simulink model "P702_NI_SoftECU"  (R2019a)
settings: Solver=ode1  StartTime=0.0  StopTime=Inf  FixedStep=0.001  RelTol=1e-3  EnableMultiTasking=on
PreLoadFcn:
  | run '.\VeriStand_BlockSet\NIVeriStandAddPaths.m'
undefined symbols (not defined in the file or in its folder): magnitude
libraries: simulink x83, simulink_extras x1
(part 70 of 76)

== system P702_NI_SoftECU/SoftECU/SRR_L/FrontLeft_SOD/SRR_FL_002/Subsystem ==
  target_pos : Inport
  sensor_pos : Inport  Port=2
  CSP : Inport  Port=3
  Abs : Abs
  Add : Sum  Inputs=++-+
  Add1 : Sum  Inputs=++-+
  Add2 : Sum  Inputs=+-
  Add3 : Sum
  Bus Selector : BusSelector  OutputSignals=SRR_L_DET_RANGE_02[m],SRR_L_DET_AZIMUTH_02[rad],SRR_L_DET_RANGE_RATE_02[m/s],SRR_L_DET_ELEVATION_02[rad]
  Bus Selector1 : BusSelector  OutputSignals=sensor_x,sensor_y,sensor_yaw
  Bus Selector2 : BusSelector  OutputSignals=c_sensor_x,c_sensor_y,c_sensor_yaw
  Constant : Constant
  Index Vector : MultiPortSwitch  DataPortOrder=Zero-based contiguous  Inputs=2  zeroidx=on
  Index Vector1 : MultiPortSwitch  DataPortOrder=Zero-based contiguous  Inputs=2  zeroidx=on
  Logical Operator : Logic  AllPortsSameDT=off  OutDataTypeStr=boolean
  Math Function : Math  Operator=magnitude^2  SaturateOnIntegerOverflow=on
  Math Function1 : Math  Operator=magnitude^2  SaturateOnIntegerOverflow=on
  Product : Product
  Product1 : Product
  Product2 : Product
  Relational Operator : RelationalOperator  Operator=<=  OutDataTypeStr=boolean  RndMeth=Simplest
  Relational Operator1 : RelationalOperator  Operator=<=  OutDataTypeStr=boolean  RndMeth=Simplest
  Sqrt : Sqrt  SaturateOnIntegerOverflow=on
  Terminator : Terminator
  atan_cal : Trigonometry  Operator=atan2
  atan_cal1 : Trigonometry  Operator=atan2
  not_valid_azimuth : Constant  Value=0
  not_valid_range : Constant  Value=-1
  random_factor : Subsystem
  random_factor1 : Subsystem
  sincal : Trigonometry
  sincal1 : Trigonometry  Operator=cos
  sincal2 : Trigonometry
  sincal3 : Trigonometry  Operator=cos
  range : Outport
  range_rate : Outport  Port=2
  azimuth : Outport  Port=3
  elevation : Outport  Port=4
  wires:
  target_pos/1 -> Bus Selector/1
  Bus Selector/1 -> random_factor/1(Range), random_factor1/1(Range), Product1/1, Product/1  "<SRR_L_DET_RANGE_02[m]>"
  Bus Selector/2 -> sincal1/1, sincal/1  "<SRR_L_DET_AZIMUTH_02[rad]>"
  sincal/1 -> Product/2
  sincal1/1 -> Product1/2
  Product/1 -> Add/1
  sensor_pos/1 -> Bus Selector1/1
  CSP/1 -> Bus Selector2/1
  Bus Selector2/1 -> Add1/2  "<c_sensor_x>"
  Bus Selector2/2 -> Add/2  "<c_sensor_y>"
  Bus Selector2/3 -> Terminator/1  "<c_sensor_yaw>"
  Bus Selector1/1 -> Add1/3  "<sensor_x>"
  Bus Selector1/2 -> Add/3  "<sensor_y>"
  Bus Selector1/3 -> Add2/2  "<sensor_yaw>"
  Product1/1 -> Add1/1
  Add/1 -> Math Function/1, atan_cal/1
  Add1/1 -> Math Function1/1, atan_cal/2
  atan_cal/1 -> Add2/1
  Math Function/1 -> Add3/1
  Math Function1/1 -> Add3/2
  Add3/1 -> Sqrt/1
  Constant/1 -> Product2/2
  Bus Selector/3 -> range_rate/1  "<SRR_L_DET_RANGE_RATE_02[m/s]>"
  Bus Selector/4 -> elevation/1  "<SRR_L_DET_ELEVATION_02[rad]>"
  Sqrt/1 -> Index Vector/3, Relational Operator/1
  Product2/1 -> Abs/1, Index Vector1/3
  Relational Operator/1 -> Logical Operator/1
  Relational Operator1/1 -> Logical Operator/2
  Index Vector/1 -> range/1
  not_valid_range/1 -> Index Vector/2
  Index Vector1/1 -> azimuth/1
  Logical Operator/1 -> Index Vector1/1, Index Vector/1
  not_valid_azimuth/1 -> Index Vector1/2
  atan_cal1/1 -> Product2/1
  sincal2/1 -> atan_cal1/1
  sincal3/1 -> atan_cal1/2
  Add2/1 -> sincal3/1, sincal2/1
  Abs/1 -> Relational Operator1/1
  [DistanceScanRange] -> Relational Operator/2
  [AngleScanRange] -> Relational Operator1/2
  random_factor/1(Rand_Error) -> Add/4
  random_factor1/1(Rand_Error) -> Add1/4

== system P702_NI_SoftECU/SoftECU/SRR_L/FrontLeft_SOD/SRR_FL_003/Subsystem ==
  target_pos : Inport
  sensor_pos : Inport  Port=2
  CSP : Inport  Port=3
  Abs : Abs
  Add : Sum  Inputs=++-+
  Add1 : Sum  Inputs=++-+
  Add2 : Sum  Inputs=+-
  Add3 : Sum
  Bus Selector : BusSelector  OutputSignals=SRR_L_DET_RANGE_03[m],SRR_L_DET_AZIMUTH_03[rad],SRR_L_DET_RANGE_RATE_03[m/s],SRR_L_DET_ELEVATION_03[rad]
  Bus Selector1 : BusSelector  OutputSignals=sensor_x,sensor_y,sensor_yaw
  Bus Selector2 : BusSelector  OutputSignals=c_sensor_x,c_sensor_y,c_sensor_yaw
  Constant : Constant
  Index Vector : MultiPortSwitch  DataPortOrder=Zero-based contiguous  Inputs=2  zeroidx=on
  Index Vector1 : MultiPortSwitch  DataPortOrder=Zero-based contiguous  Inputs=2  zeroidx=on
  Logical Operator : Logic  AllPortsSameDT=off  OutDataTypeStr=boolean
  Math Function : Math  Operator=magnitude^2  SaturateOnIntegerOverflow=on
  Math Function1 : Math  Operator=magnitude^2  SaturateOnIntegerOverflow=on
  Product : Product
  Product1 : Product
  Product2 : Product
  Relational Operator : RelationalOperator  Operator=<=  OutDataTypeStr=boolean  RndMeth=Simplest
  Relational Operator1 : RelationalOperator  Operator=<=  OutDataTypeStr=boolean  RndMeth=Simplest
  Sqrt : Sqrt  SaturateOnIntegerOverflow=on
  Terminator : Terminator
  atan_cal : Trigonometry  Operator=atan2
  atan_cal1 : Trigonometry  Operator=atan2
  not_valid_azimuth : Constant  Value=0
  not_valid_range : Constant  Value=-1
  random_factor : Subsystem
  random_factor1 : Subsystem
  sincal : Trigonometry
  sincal1 : Trigonometry  Operator=cos
  sincal2 : Trigonometry
  sincal3 : Trigonometry  Operator=cos
  range : Outport
  range_rate : Outport  Port=2
  azimuth : Outport  Port=3
  elevation : Outport  Port=4
  wires:
  random_factor1/1(Rand_Error) -> Add1/4
  random_factor/1(Rand_Error) -> Add/4
  [AngleScanRange] -> Relational Operator1/2
  [DistanceScanRange] -> Relational Operator/2
  Abs/1 -> Relational Operator1/1
  Add2/1 -> sincal2/1, sincal3/1
  sincal3/1 -> atan_cal1/2
  sincal2/1 -> atan_cal1/1
  atan_cal1/1 -> Product2/1
  not_valid_azimuth/1 -> Index Vector1/2
  Logical Operator/1 -> Index Vector/1, Index Vector1/1
  Index Vector1/1 -> azimuth/1
  not_valid_range/1 -> Index Vector/2
  Index Vector/1 -> range/1
  Relational Operator1/1 -> Logical Operator/2
  Relational Operator/1 -> Logical Operator/1
  Product2/1 -> Index Vector1/3, Abs/1
  Sqrt/1 -> Relational Operator/1, Index Vector/3
  Bus Selector/4 -> elevation/1  "<SRR_L_DET_ELEVATION_03[rad]>"
  Bus Selector/3 -> range_rate/1  "<SRR_L_DET_RANGE_RATE_03[m/s]>"
  Constant/1 -> Product2/2
  Add3/1 -> Sqrt/1
  Math Function1/1 -> Add3/2
  Math Function/1 -> Add3/1
  atan_cal/1 -> Add2/1
  Add1/1 -> atan_cal/2, Math Function1/1
  Add/1 -> atan_cal/1, Math Function/1
  Product1/1 -> Add1/1
  Bus Selector1/3 -> Add2/2  "<sensor_yaw>"
  Bus Selector1/2 -> Add/3  "<sensor_y>"
  Bus Selector1/1 -> Add1/3  "<sensor_x>"
  Bus Selector2/3 -> Terminator/1  "<c_sensor_yaw>"
  Bus Selector2/2 -> Add/2  "<c_sensor_y>"
  Bus Selector2/1 -> Add1/2  "<c_sensor_x>"
  CSP/1 -> Bus Selector2/1
  sensor_pos/1 -> Bus Selector1/1
  Product/1 -> Add/1
  sincal1/1 -> Product1/2
  sincal/1 -> Product/2
  Bus Selector/2 -> sincal/1, sincal1/1  "<SRR_L_DET_AZIMUTH_03[rad]>"
  Bus Selector/1 -> Product/1, Product1/1, random_factor1/1(Range), random_factor/1(Range)  "<SRR_L_DET_RANGE_03[m]>"
  target_pos/1 -> Bus Selector/1

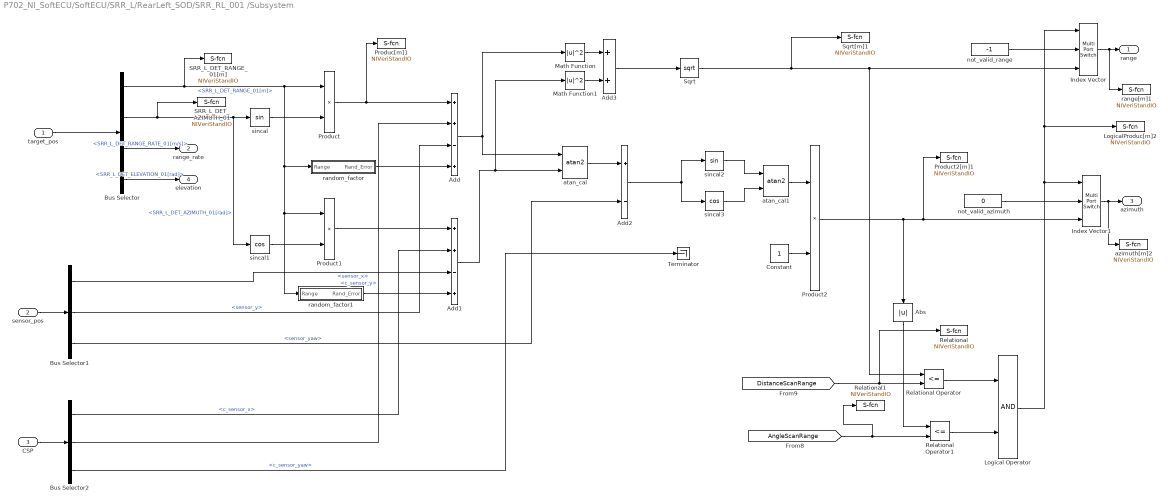
== system P702_NI_SoftECU/SoftECU/SRR_L/RearLeft_SOD/SRR_RL_001 /Subsystem ==
  target_pos : Inport
  sensor_pos : Inport  Port=2
  CSP : Inport  Port=3
  Abs : Abs
  Add : Sum  Inputs=++-+
  Add1 : Sum  Inputs=++-+
  Add2 : Sum  Inputs=+-
  Add3 : Sum
  Bus Selector : BusSelector  OutputSignals=SRR_L_DET_RANGE_01[m],SRR_L_DET_AZIMUTH_01[rad],SRR_L_DET_RANGE_RATE_01[m/s],SRR_L_DET_ELEVATION_01[rad]
  Bus Selector1 : BusSelector  OutputSignals=sensor_x,sensor_y,sensor_yaw
  Bus Selector2 : BusSelector  OutputSignals=c_sensor_x,c_sensor_y,c_sensor_yaw
  Constant : Constant
  Index Vector : MultiPortSwitch  DataPortOrder=Zero-based contiguous  Inputs=2  zeroidx=on
  Index Vector1 : MultiPortSwitch  DataPortOrder=Zero-based contiguous  Inputs=2  zeroidx=on
  Logical Operator : Logic  AllPortsSameDT=off  OutDataTypeStr=boolean
  LogicalProduc[m]2 : S-Function  Priority=4  FunctionName=NIVeriStandIO  Parameters=width dtype portnum stime stype btype  SFunctionDeploymentMode=off  EnableBusSupport=off  mask(NI VeriStand Outport){portnum=4, width=-1, stime=-1, dtype=auto, stype=auto, btype=0}
      mask prompts: portnum "Port number:"; width "Port dimensions (-1 for dynamically sized):"; stime "Sample time (-1 for inherited):"; dtype "Data type:"; stype "Signal type:"; btype "Block type:"
      mask help: Use this outport on any level of nested subsystems to allow NI VeriStand software to map signals to it.
      mask init:
      | NIVeriStandIO_init;
      settings: CopyFcn=NIVeriStand_MDL_functions('', 'IO_copy');  DeleteFcn=NIVeriStand_MDL_functions('', 'IO_delete');  MoveFcn=set_param(gcb, 'Mask', 'on');
      mask Callback portnum: NIVeriStand_MDL_functions('', 'IO_setportnum');
      mask TypeOptions dtype: auto | double | single | int8 | uint8 | int16 | uint16 | int32 | uint32 | boolean
      mask Callback dtype: NIVeriStand_MDL_functions('', 'IO_booleansignal');
      mask TypeOptions stype: auto | real | complex
      mask Display:
      | patch([-x x], [-y y], [.90980 .81960 .32156]);
      | plot([xrad -x x xrad], [yrad -y y yrad]);
      | fprintf('NI Out%d', portnum);
  Math Function : Math  Operator=magnitude^2  SaturateOnIntegerOverflow=on
  Math Function1 : Math  Operator=magnitude^2  SaturateOnIntegerOverflow=on
  Produc[m]1 : S-Function  Priority=3  FunctionName=NIVeriStandIO  Parameters=width dtype portnum stime stype btype  SFunctionDeploymentMode=off  EnableBusSupport=off  mask(NI VeriStand Outport){portnum=3, width=-1, stime=-1, dtype=auto, stype=auto, btype=0}
      mask prompts: portnum "Port number:"; width "Port dimensions (-1 for dynamically sized):"; stime "Sample time (-1 for inherited):"; dtype "Data type:"; stype "Signal type:"; btype "Block type:"
      mask help: Use this outport on any level of nested subsystems to allow NI VeriStand software to map signals to it.
      mask init:
      | NIVeriStandIO_init;
      settings: CopyFcn=NIVeriStand_MDL_functions('', 'IO_copy');  DeleteFcn=NIVeriStand_MDL_functions('', 'IO_delete');  MoveFcn=set_param(gcb, 'Mask', 'on');
      mask Callback portnum: NIVeriStand_MDL_functions('', 'IO_setportnum');
      mask TypeOptions dtype: auto | double | single | int8 | uint8 | int16 | uint16 | int32 | uint32 | boolean
      mask Callback dtype: NIVeriStand_MDL_functions('', 'IO_booleansignal');
      mask TypeOptions stype: auto | real | complex
      mask Display:
      | patch([-x x], [-y y], [.90980 .81960 .32156]);
      | plot([xrad -x x xrad], [yrad -y y yrad]);
      | fprintf('NI Out%d', portnum);
  Product : Product
  Product1 : Product
  Product2 : Product
  Product2[m]1 : S-Function  Priority=6  FunctionName=NIVeriStandIO  Parameters=width dtype portnum stime stype btype  SFunctionDeploymentMode=off  EnableBusSupport=off  mask(NI VeriStand Outport){portnum=6, width=-1, stime=-1, dtype=auto, stype=auto, btype=0}
      mask prompts: portnum "Port number:"; width "Port dimensions (-1 for dynamically sized):"; stime "Sample time (-1 for inherited):"; dtype "Data type:"; stype "Signal type:"; btype "Block type:"
      mask help: Use this outport on any level of nested subsystems to allow NI VeriStand software to map signals to it.
      mask init:
      | NIVeriStandIO_init;
      settings: CopyFcn=NIVeriStand_MDL_functions('', 'IO_copy');  DeleteFcn=NIVeriStand_MDL_functions('', 'IO_delete');  MoveFcn=set_param(gcb, 'Mask', 'on');
      mask Callback portnum: NIVeriStand_MDL_functions('', 'IO_setportnum');
      mask TypeOptions dtype: auto | double | single | int8 | uint8 | int16 | uint16 | int32 | uint32 | boolean
      mask Callback dtype: NIVeriStand_MDL_functions('', 'IO_booleansignal');
      mask TypeOptions stype: auto | real | complex
      mask Display:
      | patch([-x x], [-y y], [.90980 .81960 .32156]);
      | plot([xrad -x x xrad], [yrad -y y yrad]);
      | fprintf('NI Out%d', portnum);
  Relational : S-Function  Priority=7  FunctionName=NIVeriStandIO  Parameters=width dtype portnum stime stype btype  SFunctionDeploymentMode=off  EnableBusSupport=off  mask(NI VeriStand Outport){portnum=7, width=-1, stime=-1, dtype=auto, stype=auto, btype=0}
      mask prompts: portnum "Port number:"; width "Port dimensions (-1 for dynamically sized):"; stime "Sample time (-1 for inherited):"; dtype "Data type:"; stype "Signal type:"; btype "Block type:"
      mask help: Use this outport on any level of nested subsystems to allow NI VeriStand software to map signals to it.
      mask init:
      | NIVeriStandIO_init;
      settings: CopyFcn=NIVeriStand_MDL_functions('', 'IO_copy');  DeleteFcn=NIVeriStand_MDL_functions('', 'IO_delete');  MoveFcn=set_param(gcb, 'Mask', 'on');
      mask Callback portnum: NIVeriStand_MDL_functions('', 'IO_setportnum');
      mask TypeOptions dtype: auto | double | single | int8 | uint8 | int16 | uint16 | int32 | uint32 | boolean
      mask Callback dtype: NIVeriStand_MDL_functions('', 'IO_booleansignal');
      mask TypeOptions stype: auto | real | complex
      mask Display:
      | patch([-x x], [-y y], [.90980 .81960 .32156]);
      | plot([xrad -x x xrad], [yrad -y y yrad]);
      | fprintf('NI Out%d', portnum);
  Relational Operator : RelationalOperator  Operator=<=  OutDataTypeStr=boolean  RndMeth=Simplest
  Relational Operator1 : RelationalOperator  Operator=<=  OutDataTypeStr=boolean  RndMeth=Simplest
  Relational1 : S-Function  Priority=8  FunctionName=NIVeriStandIO  Parameters=width dtype portnum stime stype btype  SFunctionDeploymentMode=off  EnableBusSupport=off  mask(NI VeriStand Outport){portnum=8, width=-1, stime=-1, dtype=auto, stype=auto, btype=0}
      mask prompts: portnum "Port number:"; width "Port dimensions (-1 for dynamically sized):"; stime "Sample time (-1 for inherited):"; dtype "Data type:"; stype "Signal type:"; btype "Block type:"
      mask help: Use this outport on any level of nested subsystems to allow NI VeriStand software to map signals to it.
      mask init:
      | NIVeriStandIO_init;
      settings: CopyFcn=NIVeriStand_MDL_functions('', 'IO_copy');  DeleteFcn=NIVeriStand_MDL_functions('', 'IO_delete');  MoveFcn=set_param(gcb, 'Mask', 'on');
      mask Callback portnum: NIVeriStand_MDL_functions('', 'IO_setportnum');
      mask TypeOptions dtype: auto | double | single | int8 | uint8 | int16 | uint16 | int32 | uint32 | boolean
      mask Callback dtype: NIVeriStand_MDL_functions('', 'IO_booleansignal');
      mask TypeOptions stype: auto | real | complex
      mask Display:
      | patch([-x x], [-y y], [.90980 .81960 .32156]);
      | plot([xrad -x x xrad], [yrad -y y yrad]);
      | fprintf('NI Out%d', portnum);
  SRR_L_DET_AZIMUTH_01 : S-Function  Priority=2  FunctionName=NIVeriStandIO  Parameters=width dtype portnum stime stype btype  SFunctionDeploymentMode=off  EnableBusSupport=off  mask(NI VeriStand Outport){portnum=2, width=-1, stime=-1, dtype=auto, stype=auto, btype=0}
      mask prompts: portnum "Port number:"; width "Port dimensions (-1 for dynamically sized):"; stime "Sample time (-1 for inherited):"; dtype "Data type:"; stype "Signal type:"; btype "Block type:"
      mask help: Use this outport on any level of nested subsystems to allow NI VeriStand software to map signals to it.
      mask init:
      | NIVeriStandIO_init;
      settings: CopyFcn=NIVeriStand_MDL_functions('', 'IO_copy');  DeleteFcn=NIVeriStand_MDL_functions('', 'IO_delete');  MoveFcn=set_param(gcb, 'Mask', 'on');
      mask Callback portnum: NIVeriStand_MDL_functions('', 'IO_setportnum');
      mask TypeOptions dtype: auto | double | single | int8 | uint8 | int16 | uint16 | int32 | uint32 | boolean
      mask Callback dtype: NIVeriStand_MDL_functions('', 'IO_booleansignal');
      mask TypeOptions stype: auto | real | complex
      mask Display:
      | patch([-x x], [-y y], [.90980 .81960 .32156]);
      | plot([xrad -x x xrad], [yrad -y y yrad]);
      | fprintf('NI Out%d', portnum);
  SRR_L_DET_RANGE_01[m] : S-Function  Priority=1  FunctionName=NIVeriStandIO  Parameters=width dtype portnum stime stype btype  SFunctionDeploymentMode=off  EnableBusSupport=off  mask(NI VeriStand Outport){portnum=1, width=-1, stime=-1, dtype=auto, stype=auto, btype=0}
      mask prompts: portnum "Port number:"; width "Port dimensions (-1 for dynamically sized):"; stime "Sample time (-1 for inherited):"; dtype "Data type:"; stype "Signal type:"; btype "Block type:"
      mask help: Use this outport on any level of nested subsystems to allow NI VeriStand software to map signals to it.
      mask init:
      | NIVeriStandIO_init;
      settings: CopyFcn=NIVeriStand_MDL_functions('', 'IO_copy');  DeleteFcn=NIVeriStand_MDL_functions('', 'IO_delete');  MoveFcn=set_param(gcb, 'Mask', 'on');
      mask Callback portnum: NIVeriStand_MDL_functions('', 'IO_setportnum');
      mask TypeOptions dtype: auto | double | single | int8 | uint8 | int16 | uint16 | int32 | uint32 | boolean
      mask Callback dtype: NIVeriStand_MDL_functions('', 'IO_booleansignal');
      mask TypeOptions stype: auto | real | complex
      mask Display:
      | patch([-x x], [-y y], [.90980 .81960 .32156]);
      | plot([xrad -x x xrad], [yrad -y y yrad]);
      | fprintf('NI Out%d', portnum);
  Sqrt : Sqrt  SaturateOnIntegerOverflow=on
  Sqrt[m]1 : S-Function  Priority=5  FunctionName=NIVeriStandIO  Parameters=width dtype portnum stime stype btype  SFunctionDeploymentMode=off  EnableBusSupport=off  mask(NI VeriStand Outport){portnum=5, width=-1, stime=-1, dtype=auto, stype=auto, btype=0}
      mask prompts: portnum "Port number:"; width "Port dimensions (-1 for dynamically sized):"; stime "Sample time (-1 for inherited):"; dtype "Data type:"; stype "Signal type:"; btype "Block type:"
      mask help: Use this outport on any level of nested subsystems to allow NI VeriStand software to map signals to it.
      mask init:
      | NIVeriStandIO_init;
      settings: CopyFcn=NIVeriStand_MDL_functions('', 'IO_copy');  DeleteFcn=NIVeriStand_MDL_functions('', 'IO_delete');  MoveFcn=set_param(gcb, 'Mask', 'on');
      mask Callback portnum: NIVeriStand_MDL_functions('', 'IO_setportnum');
      mask TypeOptions dtype: auto | double | single | int8 | uint8 | int16 | uint16 | int32 | uint32 | boolean
      mask Callback dtype: NIVeriStand_MDL_functions('', 'IO_booleansignal');
      mask TypeOptions stype: auto | real | complex
      mask Display:
      | patch([-x x], [-y y], [.90980 .81960 .32156]);
      | plot([xrad -x x xrad], [yrad -y y yrad]);
      | fprintf('NI Out%d', portnum);
  Terminator : Terminator
  atan_cal : Trigonometry  Operator=atan2
  atan_cal1 : Trigonometry  Operator=atan2
  azimuth[m]2 : S-Function  Priority=10  FunctionName=NIVeriStandIO  Parameters=width dtype portnum stime stype btype  SFunctionDeploymentMode=off  EnableBusSupport=off  mask(NI VeriStand Outport){portnum=10, width=-1, stime=-1, dtype=auto, stype=auto, btype=0}
      mask prompts: portnum "Port number:"; width "Port dimensions (-1 for dynamically sized):"; stime "Sample time (-1 for inherited):"; dtype "Data type:"; stype "Signal type:"; btype "Block type:"
      mask help: Use this outport on any level of nested subsystems to allow NI VeriStand software to map signals to it.
      mask init:
      | NIVeriStandIO_init;
      settings: CopyFcn=NIVeriStand_MDL_functions('', 'IO_copy');  DeleteFcn=NIVeriStand_MDL_functions('', 'IO_delete');  MoveFcn=set_param(gcb, 'Mask', 'on');
      mask Callback portnum: NIVeriStand_MDL_functions('', 'IO_setportnum');
      mask TypeOptions dtype: auto | double | single | int8 | uint8 | int16 | uint16 | int32 | uint32 | boolean
      mask Callback dtype: NIVeriStand_MDL_functions('', 'IO_booleansignal');
      mask TypeOptions stype: auto | real | complex
      mask Display:
      | patch([-x x], [-y y], [.90980 .81960 .32156]);
      | plot([xrad -x x xrad], [yrad -y y yrad]);
      | fprintf('NI Out%d', portnum);
  not_valid_azimuth : Constant  Value=0
  not_valid_range : Constant  Value=-1
  random_factor : Subsystem
  random_factor1 : Subsystem
  range[m]1 : S-Function  Priority=9  FunctionName=NIVeriStandIO  Parameters=width dtype portnum stime stype btype  SFunctionDeploymentMode=off  EnableBusSupport=off  mask(NI VeriStand Outport){portnum=9, width=-1, stime=-1, dtype=auto, stype=auto, btype=0}
      mask prompts: portnum "Port number:"; width "Port dimensions (-1 for dynamically sized):"; stime "Sample time (-1 for inherited):"; dtype "Data type:"; stype "Signal type:"; btype "Block type:"
      mask help: Use this outport on any level of nested subsystems to allow NI VeriStand software to map signals to it.
      mask init:
      | NIVeriStandIO_init;
      settings: CopyFcn=NIVeriStand_MDL_functions('', 'IO_copy');  DeleteFcn=NIVeriStand_MDL_functions('', 'IO_delete');  MoveFcn=set_param(gcb, 'Mask', 'on');
      mask Callback portnum: NIVeriStand_MDL_functions('', 'IO_setportnum');
      mask TypeOptions dtype: auto | double | single | int8 | uint8 | int16 | uint16 | int32 | uint32 | boolean
      mask Callback dtype: NIVeriStand_MDL_functions('', 'IO_booleansignal');
      mask TypeOptions stype: auto | real | complex
      mask Display:
      | patch([-x x], [-y y], [.90980 .81960 .32156]);
      | plot([xrad -x x xrad], [yrad -y y yrad]);
      | fprintf('NI Out%d', portnum);
  sincal : Trigonometry
  sincal1 : Trigonometry  Operator=cos
  sincal2 : Trigonometry
  sincal3 : Trigonometry  Operator=cos
  range : Outport
  range_rate : Outport  Port=2
  azimuth : Outport  Port=3
  elevation : Outport  Port=4
  wires:
  target_pos/1 -> Bus Selector/1
  Bus Selector/1 -> SRR_L_DET_RANGE_01[m]/1, random_factor/1(Range), random_factor1/1(Range), Product1/1, Product/1  "<SRR_L_DET_RANGE_01[m]>"
  Bus Selector/2 -> SRR_L_DET_AZIMUTH_01/1, sincal1/1, sincal/1  "<SRR_L_DET_AZIMUTH_01[rad]>"
  sincal/1 -> Product/2
  sincal1/1 -> Product1/2
  sensor_pos/1 -> Bus Selector1/1
  CSP/1 -> Bus Selector2/1
  Bus Selector2/1 -> Add1/2  "<c_sensor_x>"
  Bus Selector2/2 -> Add/2  "<c_sensor_y>"
  Bus Selector2/3 -> Terminator/1  "<c_sensor_yaw>"
  Bus Selector1/1 -> Add1/3  "<sensor_x>"
  Bus Selector1/2 -> Add/3  "<sensor_y>"
  Bus Selector1/3 -> Add2/2  "<sensor_yaw>"
  Product1/1 -> Add1/1
  Add/1 -> Math Function/1, atan_cal/1
  Add1/1 -> Math Function1/1, atan_cal/2
  atan_cal/1 -> Add2/1
  Math Function/1 -> Add3/1
  Math Function1/1 -> Add3/2
  Add3/1 -> Sqrt/1
  Constant/1 -> Product2/2
  Bus Selector/3 -> range_rate/1  "<SRR_L_DET_RANGE_RATE_01[m/s]>"
  Bus Selector/4 -> elevation/1  "<SRR_L_DET_ELEVATION_01[rad]>"
  Sqrt/1 -> Sqrt[m]1/1, Index Vector/3, Relational Operator/1
  Product2/1 -> Abs/1, Product2[m]1/1, Index Vector1/3
  Relational Operator/1 -> Logical Operator/1
  Relational Operator1/1 -> Logical Operator/2
  Index Vector/1 -> range[m]1/1, range/1
  not_valid_range/1 -> Index Vector/2
  Index Vector1/1 -> azimuth[m]2/1, azimuth/1
  Logical Operator/1 -> Index Vector1/1, Index Vector/1, LogicalProduc[m]2/1
  not_valid_azimuth/1 -> Index Vector1/2
  atan_cal1/1 -> Product2/1
  sincal2/1 -> atan_cal1/1
  sincal3/1 -> atan_cal1/2
  Add2/1 -> sincal3/1, sincal2/1
  Abs/1 -> Relational Operator1/1
  [DistanceScanRange] -> Relational/1, Relational Operator/2
  [AngleScanRange] -> Relational1/1, Relational Operator1/2
  random_factor/1(Rand_Error) -> Add/4
  random_factor1/1(Rand_Error) -> Add1/4
  Product/1 -> Produc[m]1/1, Add/1

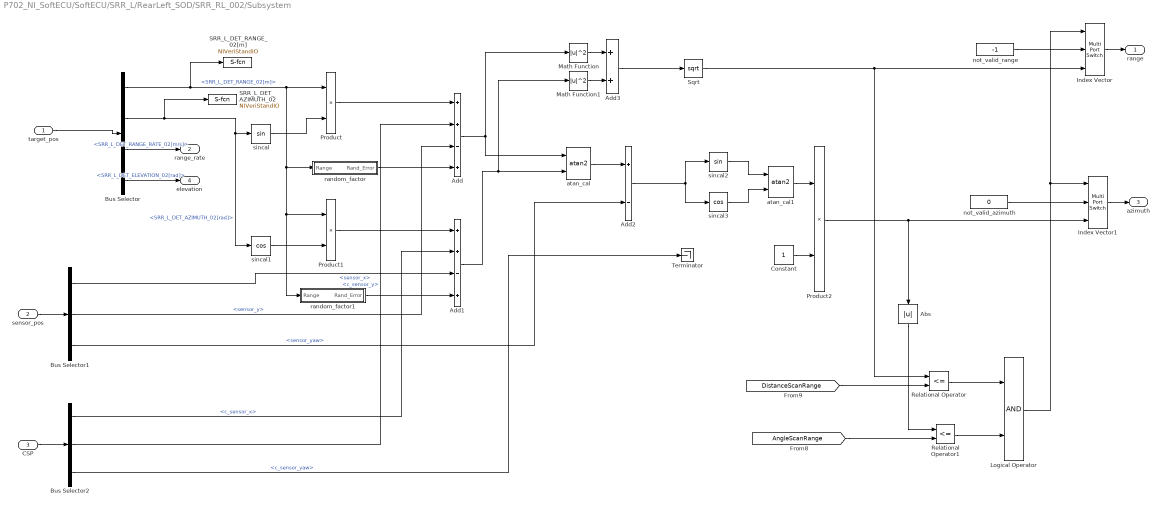
== system P702_NI_SoftECU/SoftECU/SRR_L/RearLeft_SOD/SRR_RL_002/Subsystem ==
  target_pos : Inport
  sensor_pos : Inport  Port=2
  CSP : Inport  Port=3
  Abs : Abs
  Add : Sum  Inputs=++-+
  Add1 : Sum  Inputs=++-+
  Add2 : Sum  Inputs=+-
  Add3 : Sum
  Bus Selector : BusSelector  OutputSignals=SRR_L_DET_RANGE_02[m],SRR_L_DET_AZIMUTH_02[rad],SRR_L_DET_RANGE_RATE_02[m/s],SRR_L_DET_ELEVATION_02[rad]
  Bus Selector1 : BusSelector  OutputSignals=sensor_x,sensor_y,sensor_yaw
  Bus Selector2 : BusSelector  OutputSignals=c_sensor_x,c_sensor_y,c_sensor_yaw
  Constant : Constant
  Index Vector : MultiPortSwitch  DataPortOrder=Zero-based contiguous  Inputs=2  zeroidx=on
  Index Vector1 : MultiPortSwitch  DataPortOrder=Zero-based contiguous  Inputs=2  zeroidx=on
  Logical Operator : Logic  AllPortsSameDT=off  OutDataTypeStr=boolean
  Math Function : Math  Operator=magnitude^2  SaturateOnIntegerOverflow=on
  Math Function1 : Math  Operator=magnitude^2  SaturateOnIntegerOverflow=on
  Product : Product
  Product1 : Product
  Product2 : Product
  Relational Operator : RelationalOperator  Operator=<=  OutDataTypeStr=boolean  RndMeth=Simplest
  Relational Operator1 : RelationalOperator  Operator=<=  OutDataTypeStr=boolean  RndMeth=Simplest
  SRR_L_DET_AZIMUTH_02 : S-Function  Priority=2  FunctionName=NIVeriStandIO  Parameters=width dtype portnum stime stype btype  SFunctionDeploymentMode=off  EnableBusSupport=off  mask(NI VeriStand Outport){portnum=2, width=-1, stime=-1, dtype=auto, stype=auto, btype=0}
      mask prompts: portnum "Port number:"; width "Port dimensions (-1 for dynamically sized):"; stime "Sample time (-1 for inherited):"; dtype "Data type:"; stype "Signal type:"; btype "Block type:"
      mask help: Use this outport on any level of nested subsystems to allow NI VeriStand software to map signals to it.
      mask init:
      | NIVeriStandIO_init;
      settings: CopyFcn=NIVeriStand_MDL_functions('', 'IO_copy');  DeleteFcn=NIVeriStand_MDL_functions('', 'IO_delete');  MoveFcn=set_param(gcb, 'Mask', 'on');
      mask Callback portnum: NIVeriStand_MDL_functions('', 'IO_setportnum');
      mask TypeOptions dtype: auto | double | single | int8 | uint8 | int16 | uint16 | int32 | uint32 | boolean
      mask Callback dtype: NIVeriStand_MDL_functions('', 'IO_booleansignal');
      mask TypeOptions stype: auto | real | complex
      mask Display:
      | patch([-x x], [-y y], [.90980 .81960 .32156]);
      | plot([xrad -x x xrad], [yrad -y y yrad]);
      | fprintf('NI Out%d', portnum);
  SRR_L_DET_RANGE_02[m] : S-Function  Priority=1  FunctionName=NIVeriStandIO  Parameters=width dtype portnum stime stype btype  SFunctionDeploymentMode=off  EnableBusSupport=off  mask(NI VeriStand Outport){portnum=1, width=-1, stime=-1, dtype=auto, stype=auto, btype=0}
      mask prompts: portnum "Port number:"; width "Port dimensions (-1 for dynamically sized):"; stime "Sample time (-1 for inherited):"; dtype "Data type:"; stype "Signal type:"; btype "Block type:"
      mask help: Use this outport on any level of nested subsystems to allow NI VeriStand software to map signals to it.
      mask init:
      | NIVeriStandIO_init;
      settings: CopyFcn=NIVeriStand_MDL_functions('', 'IO_copy');  DeleteFcn=NIVeriStand_MDL_functions('', 'IO_delete');  MoveFcn=set_param(gcb, 'Mask', 'on');
      mask Callback portnum: NIVeriStand_MDL_functions('', 'IO_setportnum');
      mask TypeOptions dtype: auto | double | single | int8 | uint8 | int16 | uint16 | int32 | uint32 | boolean
      mask Callback dtype: NIVeriStand_MDL_functions('', 'IO_booleansignal');
      mask TypeOptions stype: auto | real | complex
      mask Display:
      | patch([-x x], [-y y], [.90980 .81960 .32156]);
      | plot([xrad -x x xrad], [yrad -y y yrad]);
      | fprintf('NI Out%d', portnum);
  Sqrt : Sqrt  SaturateOnIntegerOverflow=on
  Terminator : Terminator
  atan_cal : Trigonometry  Operator=atan2
  atan_cal1 : Trigonometry  Operator=atan2
  not_valid_azimuth : Constant  Value=0
  not_valid_range : Constant  Value=-1
  random_factor : Subsystem
  random_factor1 : Subsystem
  sincal : Trigonometry
  sincal1 : Trigonometry  Operator=cos
  sincal2 : Trigonometry
  sincal3 : Trigonometry  Operator=cos
  range : Outport
  range_rate : Outport  Port=2
  azimuth : Outport  Port=3
  elevation : Outport  Port=4
  wires:
  random_factor1/1(Rand_Error) -> Add1/4
  random_factor/1(Rand_Error) -> Add/4
  [AngleScanRange] -> Relational Operator1/2
  [DistanceScanRange] -> Relational Operator/2
  Abs/1 -> Relational Operator1/1
  Add2/1 -> sincal2/1, sincal3/1
  sincal3/1 -> atan_cal1/2
  sincal2/1 -> atan_cal1/1
  atan_cal1/1 -> Product2/1
  not_valid_azimuth/1 -> Index Vector1/2
  Logical Operator/1 -> Index Vector/1, Index Vector1/1
  Index Vector1/1 -> azimuth/1
  not_valid_range/1 -> Index Vector/2
  Index Vector/1 -> range/1
  Relational Operator1/1 -> Logical Operator/2
  Relational Operator/1 -> Logical Operator/1
  Product2/1 -> Index Vector1/3, Abs/1
  Sqrt/1 -> Relational Operator/1, Index Vector/3
  Bus Selector/4 -> elevation/1  "<SRR_L_DET_ELEVATION_02[rad]>"
  Bus Selector/3 -> range_rate/1  "<SRR_L_DET_RANGE_RATE_02[m/s]>"
  Constant/1 -> Product2/2
  Add3/1 -> Sqrt/1
  Math Function1/1 -> Add3/2
  Math Function/1 -> Add3/1
  atan_cal/1 -> Add2/1
  Add1/1 -> atan_cal/2, Math Function1/1
  Add/1 -> atan_cal/1, Math Function/1
  Product1/1 -> Add1/1
  Bus Selector1/3 -> Add2/2  "<sensor_yaw>"
  Bus Selector1/2 -> Add/3  "<sensor_y>"
  Bus Selector1/1 -> Add1/3  "<sensor_x>"
  Bus Selector2/3 -> Terminator/1  "<c_sensor_yaw>"
  Bus Selector2/2 -> Add/2  "<c_sensor_y>"
  Bus Selector2/1 -> Add1/2  "<c_sensor_x>"
  CSP/1 -> Bus Selector2/1
  sensor_pos/1 -> Bus Selector1/1
  Product/1 -> Add/1
  sincal1/1 -> Product1/2
  sincal/1 -> Product/2
  Bus Selector/2 -> SRR_L_DET_AZIMUTH_02/1, sincal/1, sincal1/1  "<SRR_L_DET_AZIMUTH_02[rad]>"
  Bus Selector/1 -> SRR_L_DET_RANGE_02[m]/1, Product/1, Product1/1, random_factor1/1(Range), random_factor/1(Range)  "<SRR_L_DET_RANGE_02[m]>"
  target_pos/1 -> Bus Selector/1

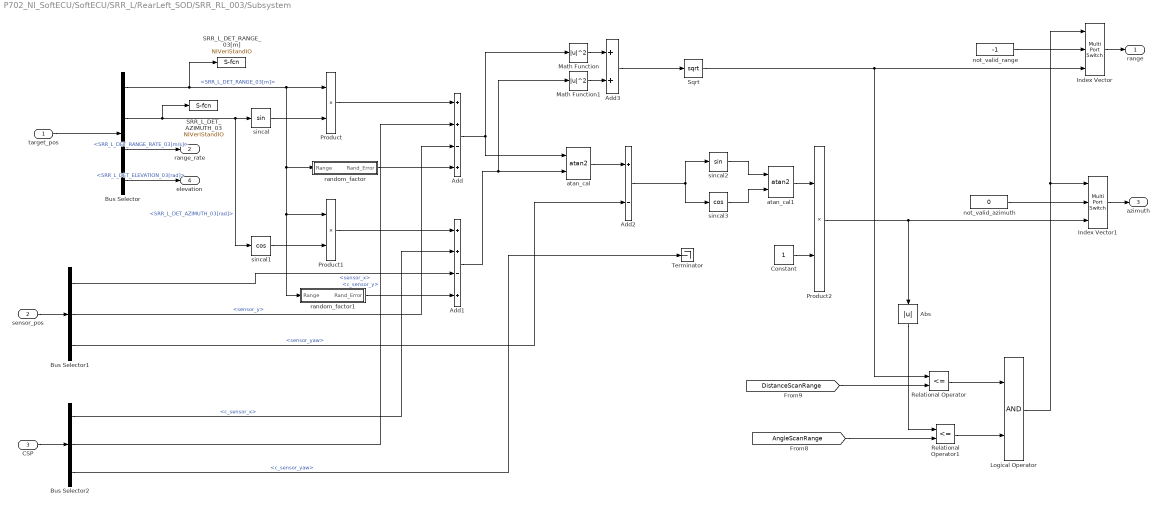
== system P702_NI_SoftECU/SoftECU/SRR_L/RearLeft_SOD/SRR_RL_003/Subsystem ==
  target_pos : Inport
  sensor_pos : Inport  Port=2
  CSP : Inport  Port=3
  Abs : Abs
  Add : Sum  Inputs=++-+
  Add1 : Sum  Inputs=++-+
  Add2 : Sum  Inputs=+-
  Add3 : Sum
  Bus Selector : BusSelector  OutputSignals=SRR_L_DET_RANGE_03[m],SRR_L_DET_AZIMUTH_03[rad],SRR_L_DET_RANGE_RATE_03[m/s],SRR_L_DET_ELEVATION_03[rad]
  Bus Selector1 : BusSelector  OutputSignals=sensor_x,sensor_y,sensor_yaw
  Bus Selector2 : BusSelector  OutputSignals=c_sensor_x,c_sensor_y,c_sensor_yaw
  Constant : Constant
  Index Vector : MultiPortSwitch  DataPortOrder=Zero-based contiguous  Inputs=2  zeroidx=on
  Index Vector1 : MultiPortSwitch  DataPortOrder=Zero-based contiguous  Inputs=2  zeroidx=on
  Logical Operator : Logic  AllPortsSameDT=off  OutDataTypeStr=boolean
  Math Function : Math  Operator=magnitude^2  SaturateOnIntegerOverflow=on
  Math Function1 : Math  Operator=magnitude^2  SaturateOnIntegerOverflow=on
  Product : Product
  Product1 : Product
  Product2 : Product
  Relational Operator : RelationalOperator  Operator=<=  OutDataTypeStr=boolean  RndMeth=Simplest
  Relational Operator1 : RelationalOperator  Operator=<=  OutDataTypeStr=boolean  RndMeth=Simplest
  SRR_L_DET_AZIMUTH_03 : S-Function  Priority=2  FunctionName=NIVeriStandIO  Parameters=width dtype portnum stime stype btype  SFunctionDeploymentMode=off  EnableBusSupport=off  mask(NI VeriStand Outport){portnum=2, width=-1, stime=-1, dtype=auto, stype=auto, btype=0}
      mask prompts: portnum "Port number:"; width "Port dimensions (-1 for dynamically sized):"; stime "Sample time (-1 for inherited):"; dtype "Data type:"; stype "Signal type:"; btype "Block type:"
      mask help: Use this outport on any level of nested subsystems to allow NI VeriStand software to map signals to it.
      mask init:
      | NIVeriStandIO_init;
      settings: CopyFcn=NIVeriStand_MDL_functions('', 'IO_copy');  DeleteFcn=NIVeriStand_MDL_functions('', 'IO_delete');  MoveFcn=set_param(gcb, 'Mask', 'on');
      mask Callback portnum: NIVeriStand_MDL_functions('', 'IO_setportnum');
      mask TypeOptions dtype: auto | double | single | int8 | uint8 | int16 | uint16 | int32 | uint32 | boolean
      mask Callback dtype: NIVeriStand_MDL_functions('', 'IO_booleansignal');
      mask TypeOptions stype: auto | real | complex
      mask Display:
      | patch([-x x], [-y y], [.90980 .81960 .32156]);
      | plot([xrad -x x xrad], [yrad -y y yrad]);
      | fprintf('NI Out%d', portnum);
  SRR_L_DET_RANGE_03[m] : S-Function  Priority=1  FunctionName=NIVeriStandIO  Parameters=width dtype portnum stime stype btype  SFunctionDeploymentMode=off  EnableBusSupport=off  mask(NI VeriStand Outport){portnum=1, width=-1, stime=-1, dtype=auto, stype=auto, btype=0}
      mask prompts: portnum "Port number:"; width "Port dimensions (-1 for dynamically sized):"; stime "Sample time (-1 for inherited):"; dtype "Data type:"; stype "Signal type:"; btype "Block type:"
      mask help: Use this outport on any level of nested subsystems to allow NI VeriStand software to map signals to it.
      mask init:
      | NIVeriStandIO_init;
      settings: CopyFcn=NIVeriStand_MDL_functions('', 'IO_copy');  DeleteFcn=NIVeriStand_MDL_functions('', 'IO_delete');  MoveFcn=set_param(gcb, 'Mask', 'on');
      mask Callback portnum: NIVeriStand_MDL_functions('', 'IO_setportnum');
      mask TypeOptions dtype: auto | double | single | int8 | uint8 | int16 | uint16 | int32 | uint32 | boolean
      mask Callback dtype: NIVeriStand_MDL_functions('', 'IO_booleansignal');
      mask TypeOptions stype: auto | real | complex
      mask Display:
      | patch([-x x], [-y y], [.90980 .81960 .32156]);
      | plot([xrad -x x xrad], [yrad -y y yrad]);
      | fprintf('NI Out%d', portnum);
  Sqrt : Sqrt  SaturateOnIntegerOverflow=on
  Terminator : Terminator
  atan_cal : Trigonometry  Operator=atan2
  atan_cal1 : Trigonometry  Operator=atan2
  not_valid_azimuth : Constant  Value=0
  not_valid_range : Constant  Value=-1
  random_factor : Subsystem
  random_factor1 : Subsystem
  sincal : Trigonometry
  sincal1 : Trigonometry  Operator=cos
  sincal2 : Trigonometry
  sincal3 : Trigonometry  Operator=cos
  range : Outport
  range_rate : Outport  Port=2
  azimuth : Outport  Port=3
  elevation : Outport  Port=4
  wires:
  target_pos/1 -> Bus Selector/1
  Bus Selector/1 -> SRR_L_DET_RANGE_03[m]/1, random_factor/1(Range), random_factor1/1(Range), Product1/1, Product/1  "<SRR_L_DET_RANGE_03[m]>"
  Bus Selector/2 -> SRR_L_DET_AZIMUTH_03/1, sincal1/1, sincal/1  "<SRR_L_DET_AZIMUTH_03[rad]>"
  sincal/1 -> Product/2
  sincal1/1 -> Product1/2
  Product/1 -> Add/1
  sensor_pos/1 -> Bus Selector1/1
  CSP/1 -> Bus Selector2/1
  Bus Selector2/1 -> Add1/2  "<c_sensor_x>"
  Bus Selector2/2 -> Add/2  "<c_sensor_y>"
  Bus Selector2/3 -> Terminator/1  "<c_sensor_yaw>"
  Bus Selector1/1 -> Add1/3  "<sensor_x>"
  Bus Selector1/2 -> Add/3  "<sensor_y>"
  Bus Selector1/3 -> Add2/2  "<sensor_yaw>"
  Product1/1 -> Add1/1
  Add/1 -> Math Function/1, atan_cal/1
  Add1/1 -> Math Function1/1, atan_cal/2
  atan_cal/1 -> Add2/1
  Math Function/1 -> Add3/1
  Math Function1/1 -> Add3/2
  Add3/1 -> Sqrt/1
  Constant/1 -> Product2/2
  Bus Selector/3 -> range_rate/1  "<SRR_L_DET_RANGE_RATE_03[m/s]>"
  Bus Selector/4 -> elevation/1  "<SRR_L_DET_ELEVATION_03[rad]>"
  Sqrt/1 -> Index Vector/3, Relational Operator/1
  Product2/1 -> Abs/1, Index Vector1/3
  Relational Operator/1 -> Logical Operator/1
  Relational Operator1/1 -> Logical Operator/2
  Index Vector/1 -> range/1
  not_valid_range/1 -> Index Vector/2
  Index Vector1/1 -> azimuth/1
  Logical Operator/1 -> Index Vector1/1, Index Vector/1
  not_valid_azimuth/1 -> Index Vector1/2
  atan_cal1/1 -> Product2/1
  sincal2/1 -> atan_cal1/1
  sincal3/1 -> atan_cal1/2
  Add2/1 -> sincal3/1, sincal2/1
  Abs/1 -> Relational Operator1/1
  [DistanceScanRange] -> Relational Operator/2
  [AngleScanRange] -> Relational Operator1/2
  random_factor/1(Rand_Error) -> Add/4
  random_factor1/1(Rand_Error) -> Add1/4

== system P702_NI_SoftECU/SoftECU/SRR_R/FrontRight_SOD/SRR_FR_001 /Subsystem ==
  target_pos : Inport
  sensor_pos : Inport  Port=2
  CSP : Inport  Port=3
  Abs : Abs
  Add : Sum  Inputs=++-+
  Add1 : Sum  Inputs=++-+
  Add2 : Sum  Inputs=+-
  Add3 : Sum
  Bus Selector : BusSelector  OutputSignals=SRR_R_DET_RANGE_01[m],SRR_R_DET_AZIMUTH_01[rad],SRR_R_DET_RANGE_RATE_01[m/s],SRR_R_DET_ELEVATION_01[rad]
  Bus Selector1 : BusSelector  OutputSignals=sensor_x,sensor_y,sensor_yaw
  Bus Selector2 : BusSelector  OutputSignals=c_sensor_x,c_sensor_y,c_sensor_yaw
  Constant : Constant
  Index Vector : MultiPortSwitch  DataPortOrder=Zero-based contiguous  Inputs=2  zeroidx=on
  Index Vector1 : MultiPortSwitch  DataPortOrder=Zero-based contiguous  Inputs=2  zeroidx=on
  Logical Operator : Logic  AllPortsSameDT=off  OutDataTypeStr=boolean
  Math Function : Math  Operator=magnitude^2  SaturateOnIntegerOverflow=on
  Math Function1 : Math  Operator=magnitude^2  SaturateOnIntegerOverflow=on
  Product : Product
  Product1 : Product
  Product2 : Product
  Relational Operator : RelationalOperator  Operator=<=  OutDataTypeStr=boolean  RndMeth=Simplest
  Relational Operator1 : RelationalOperator  Operator=<=  OutDataTypeStr=boolean  RndMeth=Simplest
  Sqrt : Sqrt  SaturateOnIntegerOverflow=on
  Terminator : Terminator
  atan_cal : Trigonometry  Operator=atan2
  atan_cal1 : Trigonometry  Operator=atan2
  not_valid_azimuth : Constant  Value=0
  not_valid_range : Constant  Value=-1
  random_factor : Subsystem
  random_factor1 : Subsystem
  sincal : Trigonometry
  sincal1 : Trigonometry  Operator=cos
  sincal2 : Trigonometry
  sincal3 : Trigonometry  Operator=cos
  range : Outport
  range_rate : Outport  Port=2
  azimuth : Outport  Port=3
  elevation : Outport  Port=4
  wires:
  random_factor1/1(Rand_Error) -> Add1/4
  random_factor/1(Rand_Error) -> Add/4
  [AngleScanRange] -> Relational Operator1/2
  [DistanceScanRange] -> Relational Operator/2
  Abs/1 -> Relational Operator1/1
  Add2/1 -> sincal2/1, sincal3/1
  sincal3/1 -> atan_cal1/2
  sincal2/1 -> atan_cal1/1
  atan_cal1/1 -> Product2/1
  not_valid_azimuth/1 -> Index Vector1/2
  Logical Operator/1 -> Index Vector/1, Index Vector1/1
  Index Vector1/1 -> azimuth/1
  not_valid_range/1 -> Index Vector/2
  Index Vector/1 -> range/1
  Relational Operator1/1 -> Logical Operator/2
  Relational Operator/1 -> Logical Operator/1
  Product2/1 -> Index Vector1/3, Abs/1
  Sqrt/1 -> Relational Operator/1, Index Vector/3
  Bus Selector/4 -> elevation/1  "<SRR_R_DET_ELEVATION_01[rad]>"
  Bus Selector/3 -> range_rate/1  "<SRR_R_DET_RANGE_RATE_01[m/s]>"
  Constant/1 -> Product2/2
  Add3/1 -> Sqrt/1
  Math Function1/1 -> Add3/2
  Math Function/1 -> Add3/1
  atan_cal/1 -> Add2/1
  Add1/1 -> atan_cal/2, Math Function1/1
  Add/1 -> atan_cal/1, Math Function/1
  Product1/1 -> Add1/1
  Bus Selector1/3 -> Add2/2  "<sensor_yaw>"
  Bus Selector1/2 -> Add/3  "<sensor_y>"
  Bus Selector1/1 -> Add1/3  "<sensor_x>"
  Bus Selector2/3 -> Terminator/1  "<c_sensor_yaw>"
  Bus Selector2/2 -> Add/2  "<c_sensor_y>"
  Bus Selector2/1 -> Add1/2  "<c_sensor_x>"
  CSP/1 -> Bus Selector2/1
  sensor_pos/1 -> Bus Selector1/1
  Product/1 -> Add/1
  sincal1/1 -> Product1/2
  sincal/1 -> Product/2
  Bus Selector/2 -> sincal/1, sincal1/1  "<SRR_R_DET_AZIMUTH_01[rad]>"
  Bus Selector/1 -> Product/1, Product1/1, random_factor1/1(Range), random_factor/1(Range)  "<SRR_R_DET_RANGE_01[m]>"
  target_pos/1 -> Bus Selector/1

== system P702_NI_SoftECU/SoftECU/SRR_R/FrontRight_SOD/SRR_FR_002/Subsystem ==
  target_pos : Inport
  sensor_pos : Inport  Port=2
  CSP : Inport  Port=3
  Abs : Abs
  Add : Sum  Inputs=++-+
  Add1 : Sum  Inputs=++-+
  Add2 : Sum  Inputs=+-
  Add3 : Sum
  Bus Selector : BusSelector  OutputSignals=SRR_R_DET_RANGE_02[m],SRR_R_DET_AZIMUTH_02[rad],SRR_R_DET_RANGE_RATE_02[m/s],SRR_R_DET_ELEVATION_02[rad]
  Bus Selector1 : BusSelector  OutputSignals=sensor_x,sensor_y,sensor_yaw
  Bus Selector2 : BusSelector  OutputSignals=c_sensor_x,c_sensor_y,c_sensor_yaw
  Constant : Constant
  Index Vector : MultiPortSwitch  DataPortOrder=Zero-based contiguous  Inputs=2  zeroidx=on
  Index Vector1 : MultiPortSwitch  DataPortOrder=Zero-based contiguous  Inputs=2  zeroidx=on
  Logical Operator : Logic  AllPortsSameDT=off  OutDataTypeStr=boolean
  Math Function : Math  Operator=magnitude^2  SaturateOnIntegerOverflow=on
  Math Function1 : Math  Operator=magnitude^2  SaturateOnIntegerOverflow=on
  Product : Product
  Product1 : Product
  Product2 : Product
  Relational Operator : RelationalOperator  Operator=<=  OutDataTypeStr=boolean  RndMeth=Simplest
  Relational Operator1 : RelationalOperator  Operator=<=  OutDataTypeStr=boolean  RndMeth=Simplest
  Sqrt : Sqrt  SaturateOnIntegerOverflow=on
  Terminator : Terminator
  atan_cal : Trigonometry  Operator=atan2
  atan_cal1 : Trigonometry  Operator=atan2
  not_valid_azimuth : Constant  Value=0
  not_valid_range : Constant  Value=-1
  random_factor : Subsystem
  random_factor1 : Subsystem
  sincal : Trigonometry
  sincal1 : Trigonometry  Operator=cos
  sincal2 : Trigonometry
  sincal3 : Trigonometry  Operator=cos
  range : Outport
  range_rate : Outport  Port=2
  azimuth : Outport  Port=3
  elevation : Outport  Port=4
  wires:
  target_pos/1 -> Bus Selector/1
  Bus Selector/1 -> random_factor/1(Range), random_factor1/1(Range), Product1/1, Product/1  "<SRR_R_DET_RANGE_02[m]>"
  Bus Selector/2 -> sincal1/1, sincal/1  "<SRR_R_DET_AZIMUTH_02[rad]>"
  sincal/1 -> Product/2
  sincal1/1 -> Product1/2
  Product/1 -> Add/1
  sensor_pos/1 -> Bus Selector1/1
  CSP/1 -> Bus Selector2/1
  Bus Selector2/1 -> Add1/2  "<c_sensor_x>"
  Bus Selector2/2 -> Add/2  "<c_sensor_y>"
  Bus Selector2/3 -> Terminator/1  "<c_sensor_yaw>"
  Bus Selector1/1 -> Add1/3  "<sensor_x>"
  Bus Selector1/2 -> Add/3  "<sensor_y>"
  Bus Selector1/3 -> Add2/2  "<sensor_yaw>"
  Product1/1 -> Add1/1
  Add/1 -> Math Function/1, atan_cal/1
  Add1/1 -> Math Function1/1, atan_cal/2
  atan_cal/1 -> Add2/1
  Math Function/1 -> Add3/1
  Math Function1/1 -> Add3/2
  Add3/1 -> Sqrt/1
  Constant/1 -> Product2/2
  Bus Selector/3 -> range_rate/1  "<SRR_R_DET_RANGE_RATE_02[m/s]>"
  Bus Selector/4 -> elevation/1  "<SRR_R_DET_ELEVATION_02[rad]>"
  Sqrt/1 -> Index Vector/3, Relational Operator/1
  Product2/1 -> Abs/1, Index Vector1/3
  Relational Operator/1 -> Logical Operator/1
  Relational Operator1/1 -> Logical Operator/2
  Index Vector/1 -> range/1
  not_valid_range/1 -> Index Vector/2
  Index Vector1/1 -> azimuth/1
  Logical Operator/1 -> Index Vector1/1, Index Vector/1
  not_valid_azimuth/1 -> Index Vector1/2
  atan_cal1/1 -> Product2/1
  sincal2/1 -> atan_cal1/1
  sincal3/1 -> atan_cal1/2
  Add2/1 -> sincal3/1, sincal2/1
  Abs/1 -> Relational Operator1/1
  [DistanceScanRange] -> Relational Operator/2
  [AngleScanRange] -> Relational Operator1/2
  random_factor/1(Rand_Error) -> Add/4
  random_factor1/1(Rand_Error) -> Add1/4

== system P702_NI_SoftECU/SoftECU/SRR_R/FrontRight_SOD/SRR_FR_003/Subsystem ==
  target_pos : Inport
  sensor_pos : Inport  Port=2
  CSP : Inport  Port=3
  Abs : Abs
  Add : Sum  Inputs=++-+
  Add1 : Sum  Inputs=++-+
  Add2 : Sum  Inputs=+-
  Add3 : Sum
  Bus Selector : BusSelector  OutputSignals=SRR_R_DET_RANGE_03[m],SRR_R_DET_AZIMUTH_03[rad],SRR_R_DET_RANGE_RATE_03[m/s],SRR_R_DET_ELEVATION_03[rad]
  Bus Selector1 : BusSelector  OutputSignals=sensor_x,sensor_y,sensor_yaw
  Bus Selector2 : BusSelector  OutputSignals=c_sensor_x,c_sensor_y,c_sensor_yaw
  Constant : Constant
  Index Vector : MultiPortSwitch  DataPortOrder=Zero-based contiguous  Inputs=2  zeroidx=on
  Index Vector1 : MultiPortSwitch  DataPortOrder=Zero-based contiguous  Inputs=2  zeroidx=on
  Logical Operator : Logic  AllPortsSameDT=off  OutDataTypeStr=boolean
  Math Function : Math  Operator=magnitude^2  SaturateOnIntegerOverflow=on
  Math Function1 : Math  Operator=magnitude^2  SaturateOnIntegerOverflow=on
  Product : Product
  Product1 : Product
  Product2 : Product
  Relational Operator : RelationalOperator  Operator=<=  OutDataTypeStr=boolean  RndMeth=Simplest
  Relational Operator1 : RelationalOperator  Operator=<=  OutDataTypeStr=boolean  RndMeth=Simplest
  Sqrt : Sqrt  SaturateOnIntegerOverflow=on
  Terminator : Terminator
  atan_cal : Trigonometry  Operator=atan2
  atan_cal1 : Trigonometry  Operator=atan2
  not_valid_azimuth : Constant  Value=0
  not_valid_range : Constant  Value=-1
  random_factor : Subsystem
  random_factor1 : Subsystem
  sincal : Trigonometry
  sincal1 : Trigonometry  Operator=cos
  sincal2 : Trigonometry
  sincal3 : Trigonometry  Operator=cos
  range : Outport
  range_rate : Outport  Port=2
  azimuth : Outport  Port=3
  elevation : Outport  Port=4
  wires:
  random_factor1/1(Rand_Error) -> Add1/4
  random_factor/1(Rand_Error) -> Add/4
  [AngleScanRange] -> Relational Operator1/2
  [DistanceScanRange] -> Relational Operator/2
  Abs/1 -> Relational Operator1/1
  Add2/1 -> sincal2/1, sincal3/1
  sincal3/1 -> atan_cal1/2
  sincal2/1 -> atan_cal1/1
  atan_cal1/1 -> Product2/1
  not_valid_azimuth/1 -> Index Vector1/2
  Logical Operator/1 -> Index Vector/1, Index Vector1/1
  Index Vector1/1 -> azimuth/1
  not_valid_range/1 -> Index Vector/2
  Index Vector/1 -> range/1
  Relational Operator1/1 -> Logical Operator/2
  Relational Operator/1 -> Logical Operator/1
  Product2/1 -> Index Vector1/3, Abs/1
  Sqrt/1 -> Relational Operator/1, Index Vector/3
  Bus Selector/4 -> elevation/1  "<SRR_R_DET_ELEVATION_03[rad]>"
  Bus Selector/3 -> range_rate/1  "<SRR_R_DET_RANGE_RATE_03[m/s]>"
  Constant/1 -> Product2/2
  Add3/1 -> Sqrt/1
  Math Function1/1 -> Add3/2
  Math Function/1 -> Add3/1
  atan_cal/1 -> Add2/1
  Add1/1 -> atan_cal/2, Math Function1/1
  Add/1 -> atan_cal/1, Math Function/1
  Product1/1 -> Add1/1
  Bus Selector1/3 -> Add2/2  "<sensor_yaw>"
  Bus Selector1/2 -> Add/3  "<sensor_y>"
  Bus Selector1/1 -> Add1/3  "<sensor_x>"
  Bus Selector2/3 -> Terminator/1  "<c_sensor_yaw>"
  Bus Selector2/2 -> Add/2  "<c_sensor_y>"
  Bus Selector2/1 -> Add1/2  "<c_sensor_x>"
  CSP/1 -> Bus Selector2/1
  sensor_pos/1 -> Bus Selector1/1
  Product/1 -> Add/1
  sincal1/1 -> Product1/2
  sincal/1 -> Product/2
  Bus Selector/2 -> sincal/1, sincal1/1  "<SRR_R_DET_AZIMUTH_03[rad]>"
  Bus Selector/1 -> Product/1, Product1/1, random_factor1/1(Range), random_factor/1(Range)  "<SRR_R_DET_RANGE_03[m]>"
  target_pos/1 -> Bus Selector/1

== system P702_NI_SoftECU/SoftECU/SRR_R/RearRight_SOD/SRR_RR_001 /Subsystem ==
  target_pos : Inport
  sensor_pos : Inport  Port=2
  CSP : Inport  Port=3
  Abs : Abs
  Add : Sum  Inputs=++-+
  Add1 : Sum  Inputs=++-+
  Add2 : Sum  Inputs=+-
  Add3 : Sum
  Bus Selector : BusSelector  OutputSignals=SRR_R_DET_RANGE_01[m],SRR_R_DET_AZIMUTH_01[rad],SRR_R_DET_RANGE_RATE_01[m/s],SRR_R_DET_ELEVATION_01[rad]
  Bus Selector1 : BusSelector  OutputSignals=sensor_x,sensor_y,sensor_yaw
  Bus Selector2 : BusSelector  OutputSignals=c_sensor_x,c_sensor_y,c_sensor_yaw
  Constant : Constant
  Index Vector : MultiPortSwitch  DataPortOrder=Zero-based contiguous  Inputs=2  zeroidx=on
  Index Vector1 : MultiPortSwitch  DataPortOrder=Zero-based contiguous  Inputs=2  zeroidx=on
  Logical Operator : Logic  AllPortsSameDT=off  OutDataTypeStr=boolean
  Math Function : Math  Operator=magnitude^2  SaturateOnIntegerOverflow=on
  Math Function1 : Math  Operator=magnitude^2  SaturateOnIntegerOverflow=on
  Product : Product
  Product1 : Product
  Product2 : Product
  Relational Operator : RelationalOperator  Operator=<=  OutDataTypeStr=boolean  RndMeth=Simplest
  Relational Operator1 : RelationalOperator  Operator=<=  OutDataTypeStr=boolean  RndMeth=Simplest
  Sqrt : Sqrt  SaturateOnIntegerOverflow=on
  Terminator : Terminator
  atan_cal : Trigonometry  Operator=atan2
  atan_cal1 : Trigonometry  Operator=atan2
  not_valid_azimuth : Constant  Value=0
  not_valid_range : Constant  Value=-1
  random_factor : Subsystem
  random_factor1 : Subsystem
  sincal : Trigonometry
  sincal1 : Trigonometry  Operator=cos
  sincal2 : Trigonometry
  sincal3 : Trigonometry  Operator=cos
  range : Outport
  range_rate : Outport  Port=2
  azimuth : Outport  Port=3
  elevation : Outport  Port=4
  wires:
  target_pos/1 -> Bus Selector/1
  Bus Selector/1 -> random_factor/1(Range), random_factor1/1(Range), Product1/1, Product/1  "<SRR_R_DET_RANGE_01[m]>"
  Bus Selector/2 -> sincal1/1, sincal/1  "<SRR_R_DET_AZIMUTH_01[rad]>"
  sincal/1 -> Product/2
  sincal1/1 -> Product1/2
  Product/1 -> Add/1
  sensor_pos/1 -> Bus Selector1/1
  CSP/1 -> Bus Selector2/1
  Bus Selector2/1 -> Add1/2  "<c_sensor_x>"
  Bus Selector2/2 -> Add/2  "<c_sensor_y>"
  Bus Selector2/3 -> Terminator/1  "<c_sensor_yaw>"
  Bus Selector1/1 -> Add1/3  "<sensor_x>"
  Bus Selector1/2 -> Add/3  "<sensor_y>"
  Bus Selector1/3 -> Add2/2  "<sensor_yaw>"
  Product1/1 -> Add1/1
  Add/1 -> Math Function/1, atan_cal/1
  Add1/1 -> Math Function1/1, atan_cal/2
  atan_cal/1 -> Add2/1
  Math Function/1 -> Add3/1
  Math Function1/1 -> Add3/2
  Add3/1 -> Sqrt/1
  Constant/1 -> Product2/2
  Bus Selector/3 -> range_rate/1  "<SRR_R_DET_RANGE_RATE_01[m/s]>"
  Bus Selector/4 -> elevation/1  "<SRR_R_DET_ELEVATION_01[rad]>"
  Sqrt/1 -> Index Vector/3, Relational Operator/1
  Product2/1 -> Abs/1, Index Vector1/3
  Relational Operator/1 -> Logical Operator/1
  Relational Operator1/1 -> Logical Operator/2
  Index Vector/1 -> range/1
  not_valid_range/1 -> Index Vector/2
  Index Vector1/1 -> azimuth/1
  Logical Operator/1 -> Index Vector1/1, Index Vector/1
  not_valid_azimuth/1 -> Index Vector1/2
  atan_cal1/1 -> Product2/1
  sincal2/1 -> atan_cal1/1
  sincal3/1 -> atan_cal1/2
  Add2/1 -> sincal3/1, sincal2/1
  Abs/1 -> Relational Operator1/1
  [DistanceScanRange] -> Relational Operator/2
  [AngleScanRange] -> Relational Operator1/2
  random_factor/1(Rand_Error) -> Add/4
  random_factor1/1(Rand_Error) -> Add1/4
